simulink model "b"  (R2023b)
settings: Solver=VariableStepAuto  StartTime=0.0  StopTime=25.00  RelTol=1e-3
settings Model: Creator=Administrator  LastModifiedBy=s.sh
settings SolverCC: AlgebraicLoopSolver=TrustRegion
settings DataIOCC: ReturnWorkspaceOutputs=off
settings DebuggingCC: UnconnectedInputMsg=warning  UnconnectedOutputMsg=warning  UnconnectedLineMsg=warning  ArithmeticOperatorsInVariantConditions=warning
settings ModelReferenceCC: EnableRefExpFcnMdlSchedulingChecks=on
settings SFSimCC: SimUseLocalCustomCode=off  CustomCodeUndefinedFunction=UseInterfaceOnly
settings RTWCC: RTWUseLocalCustomCode=off

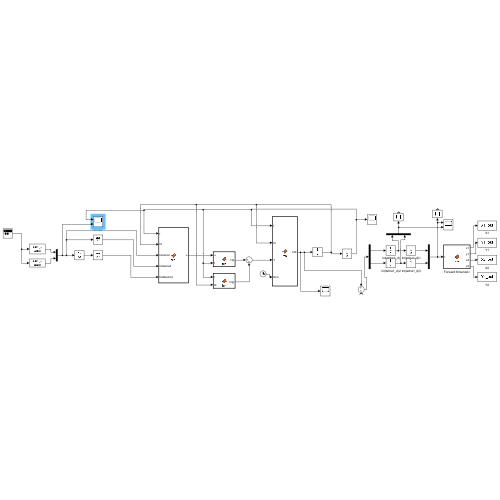
[thumbnail: Simulink's stored preview of the top-level diagram]
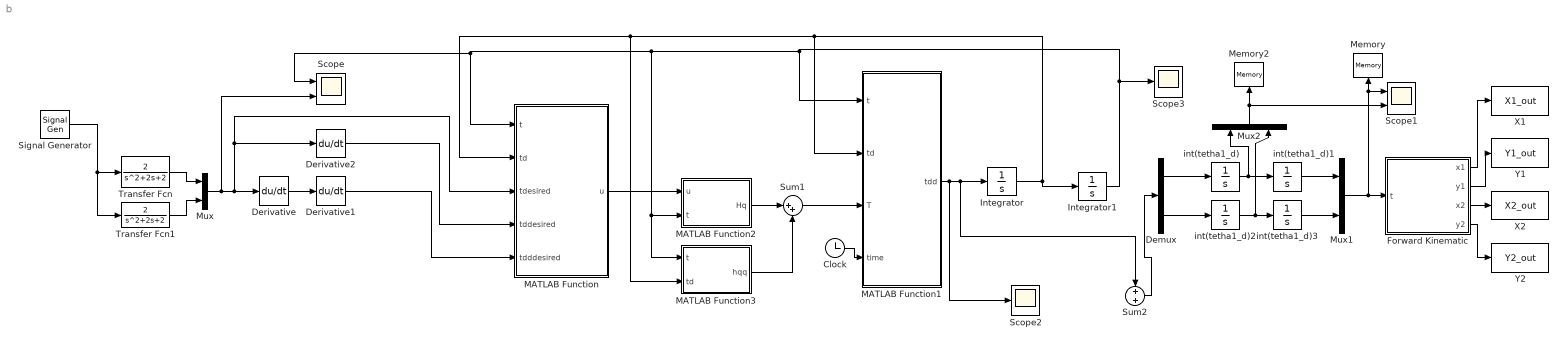
== system b ==
   int(tetha1_d){,1..3} (4 alike) : Integrator
  Clock : Clock
  Demux : Demux  Outputs=2
  Derivative : Derivative
  Derivative1 : Derivative
  Derivative2 : Derivative
  Forward Kinematic : MATLAB Function  TreatAsAtomicUnit=on
  Integrator : Integrator
  Integrator1 : Integrator
  MATLAB Function : MATLAB Function  TreatAsAtomicUnit=on
  MATLAB Function1 : MATLAB Function  TreatAsAtomicUnit=on
  MATLAB Function2 : MATLAB Function  TreatAsAtomicUnit=on
  MATLAB Function3 : MATLAB Function  TreatAsAtomicUnit=on
  Memory : Memory  InitialCondition=[0 0]
  Memory2 : Memory  InitialCondition=[0 0]
  Mux : Mux  Inputs=2
  Mux1 : Mux  Inputs=2
  Mux2 : Mux  Inputs=2
  Scope : Scope  NumInputPorts=2
  Scope1 : Scope  NumInputPorts=2
  Scope2 : Scope
  Scope3 : Scope
  Signal Generator : SignalGenerator  Amplitude=4  Frequency=pi  Units=rad/sec
  Sum1 : Sum  Inputs=|++
  Sum2 : Sum  Inputs=+|+
  Transfer Fcn : TransferFcn  Numerator=[2]  Denominator=[1 2 2]
  Transfer Fcn1 : TransferFcn  Numerator=[2]  Denominator=[1 2 2]
  X1 : ToWorkspace  VariableName=X1_out  SaveFormat=Structure With Time  SampleTime=-1
  X2 : ToWorkspace  VariableName=X2_out  SaveFormat=Structure With Time  SampleTime=-1
  Y1 : ToWorkspace  VariableName=Y1_out  SaveFormat=Structure With Time  SampleTime=-1
  Y2 : ToWorkspace  VariableName=Y2_out  SaveFormat=Structure With Time  SampleTime=-1
  wires:
  MATLAB Function1/1(tdd) -> Scope2/1, Sum2/1, Integrator/1
  Signal Generator/1 -> Transfer Fcn1/1, Transfer Fcn/1
  Mux/1 -> Derivative2/1, MATLAB Function/3(tdesired), Derivative/1, Scope/2
  Derivative/1 -> Derivative1/1
  Transfer Fcn/1 -> Mux/1
  Integrator/1 -> Integrator1/1, MATLAB Function1/2(td), MATLAB Function/2(td), MATLAB Function3/2(td)
  Transfer Fcn1/1 -> Mux/2
  MATLAB Function/1(u) -> MATLAB Function2/1(u)
  Clock/1 -> MATLAB Function1/4(time)
  MATLAB Function2/1(Hq) -> Sum1/1
  MATLAB Function3/1(hqq) -> Sum1/2
  Sum1/1 -> MATLAB Function1/3(T)
  Derivative1/1 -> MATLAB Function/5(tdddesired)
  Derivative2/1 -> MATLAB Function/4(tddesired)
  Integrator1/1 -> Scope3/1, MATLAB Function3/1(t), MATLAB Function2/2(t), Scope/1, MATLAB Function/1(t), MATLAB Function1/1(t)
  Demux/2 -> " int(tetha1_d)2"/1
  Mux2/1 -> Scope1/2, Memory2/1
  Forward Kinematic/1(x1) -> X1/1
  Forward Kinematic/4(y2) -> Y2/1
  Forward Kinematic/2(y1) -> Y1/1
  Forward Kinematic/3(x2) -> X2/1
  " int(tetha1_d)1"/1 -> Mux1/1
  " int(tetha1_d)2"/1 -> Mux2/2, " int(tetha1_d)3"/1
  Mux1/1 -> Scope1/1, Memory/1, Forward Kinematic/1(t)
  " int(tetha1_d)3"/1 -> Mux1/2
  Demux/1 -> " int(tetha1_d)"/1
  Sum2/1 -> Demux/1
  " int(tetha1_d)"/1 -> Mux2/1, " int(tetha1_d)1"/1

== matlab function b/MATLAB Function1 ==
  data: t input; td input; tdd output; T input; time input
function tdd = fcn(t, td, T , time)

tdd =[0;0];

d = 20 * sin(pi*time);

m1 = 1;
m2 = 1;
l1 = 1;
lc1 = 0.5;
l2 = 1;
lc2 = 0.5;
g = 9.81;

H11 = m1*lc1^2 + l1 + m2*(l1^2+lc2^2+2*l1*lc2*cos(t(2)))+l2;
H22 = m2*lc2^2 + l2;
H12 = m2*l1*lc2*cos(t(2)) + m2*lc2^2 + l2;
H21 = m2*l1*lc2*cos(t(2)) + m2*lc2^2 + l2;

H = [H11 H12; H21 H22];
h = m2*l1*lc2*sin(t(2));
g1 = m1*lc1*g*cos(t(1)) + m2*g*(lc2*cos(t(1)+t(2))+l1*cos(t(1)));
g2 = m2*lc2*g*cos(t(1)+t(2));
tdd = inv(H)*(T - [-h*td(2) -h*td(1)-h*td(2); h*td(1) 0]*[td(1); td(2)]-[g1; g2] + d);

== matlab function b/MATLAB Function ==
  data: t input; td input; u output; tdesired input; tddesired input; tdddesired input
function u = fcn(t, td, tdesired, tddesired, tdddesired)

KD = 20;
KP = 100;
tetha_tilted = t - tdesired;
tetha_d_tilted = td - tddesired;
u = tdddesired-(KD*(tetha_d_tilted))-(KP*(tetha_tilted));

== matlab function b/MATLAB Function2 ==
  data: u input; Hq output; t input
function Hq = fcn(u, t)
Hq=[0;0];
m1 = 1;
m2 = 1;
l1 = 1;
lc1 = 0.5;
l2 = 1;
lc2 = 0.5;
g = 9.81;

H11 = m1*lc1^2 + l1 + m2*(l1^2+lc2^2+2*l1*lc2*cos(t(2)))+l2;
H22 = m2*lc2^2 + l2;
H12 = m2*l1*lc2*cos(t(2)) + m2*lc2^2 + l2;
H21 = m2*l1*lc2*cos(t(2)) + m2*lc2^2 + l2;

H = [H11 H12; H21 H22];

Hq = H*u;

== matlab function b/MATLAB Function3 ==
  data: t input; hqq output; td input
function hqq = fcn(t, td)

hqq = [0;0];
t1=t(1);
t2=t(2);
td1=td(1);
td2=td(2);

m1 = 1;
m2 = 1;
l1 = 1;
lc1 = 0.5;
l2 = 1;
lc2 = 0.5;
h = m2*l1*lc2*sin(t(2));
g = 9.81;

g1 = m1*lc1*g*cos(t1) + m2*g*(lc2*cos(t1+t2)+l1*cos(t1));
g2 = m2*lc2*g*cos(t1+t2);

hqq = [-h*td2 -h*td1-h*td2; h*td1 0]*[td1; td2]+[g1; g2];

== matlab function b/Forward Kinematic ==
  data: t input; x1 output; y1 output; x2 output; y2 output

function [x1,y1,x2,y2] = fcn(t)
m1 = 1;
m2 = 1;
l1 = 1;
lc1 = 0.5;
l2 = 1;
lc2 = 0.5;
g = 9.81;
% Joint 2 location
x1 = l1*cos(t(1));
y1 = l1*sin(t(1));
% Joint 3 location
x2 = l1*cos(t(1))+l2*cos(t(1)+t(2));
y2 = l1*sin(t(1))+l2*sin(t(1)+t(2));
